simulink model "DSF_A3"  (R2022b)
settings: configuration reference "CommonModelConfiguration" (kept outside this file)
undefined symbols (not defined in the file or in its folder): AccSts1, AdjSpdLimnMsg1, AdjSpdLimnSts2, AdjSpdLimnWarnCoding, AsyLaneChgPsbl1, AsyLaneChgSts2, AsyLaneChgTyp2, AvlStsForAsyLaneChg, AvlStsForLatAutDrv5, AvlStsForLongAutDrv4, AvlStsForSteerSpprt1, Boolean, CarModSts1, CllsnAidPostEve3, CrsCtrlrMsg1, CrsCtrlrSts1, CrvtSpdAdj2, CtryForRoadSgn1, DrvrSpprtFct, E_CommonStatus, E_DSF_Event, E_DSF_Messages, E_DSF_Value, FctSts2, FctStsSpdCtrl, HmiAutnmsSts1, LaneDetnSts1, LCFG_SetSpeedMinKPH, LCFG_SetSpeedMinKPH_A3, LvlWarn1, MplLvlVisWarn1, NoYesCrit1, OffOnNotAvlSrvRqrd, OnOff1, PsdNotPsd, SetSpdSelnForAutDrv1, SpdAdjmtEveForAutDrv, SpdUnit1, SteerIntvSts1, SteerStsForAutDrv3, SteerWarnReqForAutDrv1, SteerWarnSts1, UndrtknPrevnWarnReq, UsgModSts1, VehDetd1, VehSpdIndcdUnit, VisWarnReq1
libraries: simulink x127
(part 2 of 3)

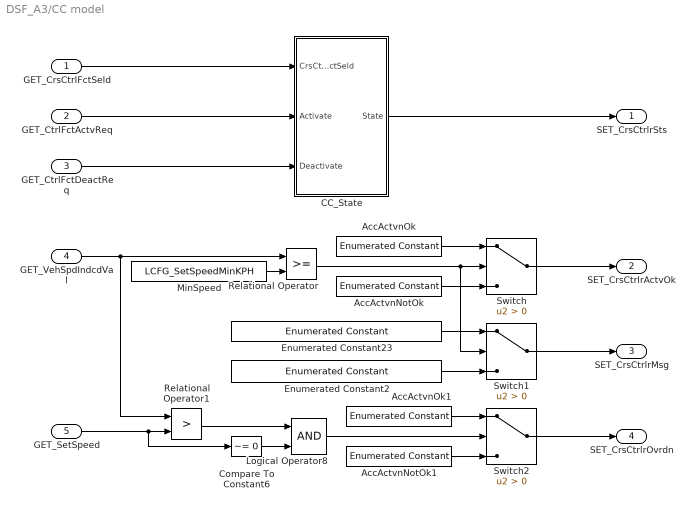
== system DSF_A3/CC model ==
  GET_CrsCtrlFctSeld : Inport
  GET_CtrlFctActvReq : Inport  Port=2
  GET_CtrlFctDeactReq : Inport  Port=3
  GET_VehSpdIndcdVal : Inport  Port=4
  GET_SetSpeed : Inport  Port=5
  AccActvnNotOk : simulink/Sources/Enumerated Constant  OutDataTypeStr=Enum: OnOff1  Value=OnOff1.OnOff1_Off  SampleTime=inf
  AccActvnNotOk1 : simulink/Sources/Enumerated Constant  OutDataTypeStr=Enum: OnOff1  Value=OnOff1.OnOff1_Off  SampleTime=inf
  AccActvnOk : simulink/Sources/Enumerated Constant  OutDataTypeStr=Enum: OnOff1  Value=OnOff1.OnOff1_On  SampleTime=inf
  AccActvnOk1 : simulink/Sources/Enumerated Constant  OutDataTypeStr=Enum: OnOff1  Value=OnOff1.OnOff1_On  SampleTime=inf
  CC_State : Stateflow chart  TreatAsAtomicUnit=on
  Compare To Constant6 : simulink/Logic and Bit Operations/Compare To Constant  relop=~=  const=0  OutDataTypeStr=boolean
  Enumerated Constant2 : simulink/Sources/Enumerated Constant  OutDataTypeStr=Enum: CrsCtrlrMsg1  Value=CrsCtrlrMsg1.CrsCtrlrMsg1_SpdLoLimExcdd  SampleTime=inf
  Enumerated Constant23 : simulink/Sources/Enumerated Constant  OutDataTypeStr=Enum: CrsCtrlrMsg1  Value=CrsCtrlrMsg1.CrsCtrlrMsg1_NoMsg  SampleTime=inf
  Logical Operator8 : Logic  AllPortsSameDT=off  OutDataTypeStr=boolean
  MinSpeed : Constant  Value=LCFG_SetSpeedMinKPH
  Relational Operator : RelationalOperator  OutDataTypeStr=boolean  RndMeth=Simplest  InputSameDT=off
  Relational Operator1 : RelationalOperator  Operator=>  OutDataTypeStr=boolean  RndMeth=Simplest  InputSameDT=off
  Switch : Switch  Criteria=u2 > Threshold  SaturateOnIntegerOverflow=off  InputSameDT=off
  Switch1 : Switch  Criteria=u2 > Threshold  SaturateOnIntegerOverflow=off  InputSameDT=off
  Switch2 : Switch  Criteria=u2 > Threshold  SaturateOnIntegerOverflow=off  InputSameDT=off
  SET_CrsCtrlrSts : Outport
  SET_CrsCtrlrActvOk : Outport  Port=2
  SET_CrsCtrlrMsg : Outport  Port=3
  SET_CrsCtrlrOvrdn : Outport  Port=4
  wires:
  AccActvnOk/1 -> Switch/1
  Relational Operator/1 -> Switch1/2, Switch/2
  MinSpeed/1 -> Relational Operator/2
  GET_VehSpdIndcdVal/1 -> Relational Operator1/1, Relational Operator/1
  Switch/1 -> SET_CrsCtrlrActvOk/1
  AccActvnNotOk/1 -> Switch/3
  Switch1/1 -> SET_CrsCtrlrMsg/1
  Enumerated Constant23/1 -> Switch1/1
  Enumerated Constant2/1 -> Switch1/3
  Switch2/1 -> SET_CrsCtrlrOvrdn/1
  AccActvnOk1/1 -> Switch2/1
  AccActvnNotOk1/1 -> Switch2/3
  Relational Operator1/1 -> Logical Operator8/1
  GET_SetSpeed/1 -> Compare To Constant6/1, Relational Operator1/2
  Logical Operator8/1 -> Switch2/2
  Compare To Constant6/1 -> Logical Operator8/2
  CC_State/1(State) -> SET_CrsCtrlrSts/1
  GET_CrsCtrlFctSeld/1 -> CC_State/1(CrsCtrlFctSeld)
  GET_CtrlFctActvReq/1 -> CC_State/2(Activate)
  GET_CtrlFctDeactReq/1 -> CC_State/3(Deactivate)

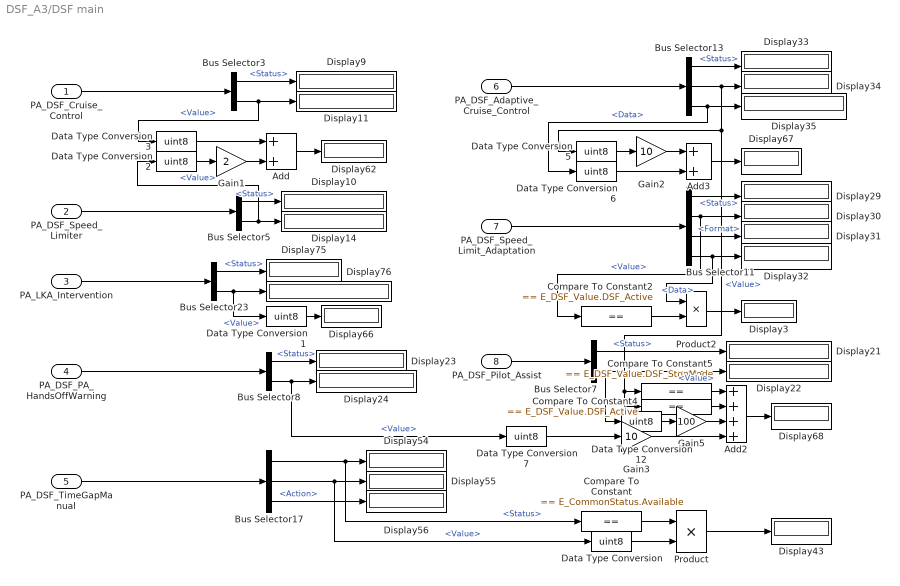
== system DSF_A3/DSF main ==
  PA_DSF_Cruise_Control : Inport
  PA_DSF_Speed_Limiter : Inport  Port=2
  PA_LKA_Intervention : Inport  Port=3
  PA_DSF_PA_HandsOffWarning : Inport  Port=4
  PA_DSF_TimeGapManual : Inport  Port=5
  PA_DSF_Adaptive_Cruise_Control : Inport  Port=6
  PA_DSF_Speed_Limit_Adaptation : Inport  Port=7
  PA_DSF_Pilot_Assist : Inport  Port=8
  Add : Sum
  Add2 : Sum  Inputs=++++
  Add3 : Sum
  Bus Selector11 : BusSelector  OutputSignals=Status,Value,Format,Data
  Bus Selector13 : BusSelector  OutputSignals=Status,Value,Data
  Bus Selector17 : BusSelector  OutputSignals=Status,Value,Action
  Bus Selector{3,5,7..8,23} (5 alike) : BusSelector  OutputSignals=Status,Value
  Compare To Constant : simulink/Logic and Bit Operations/Compare To Constant  relop===  const=E_CommonStatus.Available  OutDataTypeStr=boolean
  Compare To Constant2 : simulink/Logic and Bit Operations/Compare To Constant  relop===  const=E_DSF_Value.DSF_Active  OutDataTypeStr=boolean
  Compare To Constant4 : simulink/Logic and Bit Operations/Compare To Constant  relop===  const=E_DSF_Value.DSF_Active  OutDataTypeStr=boolean
  Compare To Constant5 : simulink/Logic and Bit Operations/Compare To Constant  relop===  const=E_DSF_Value.DSF_StopMode  OutDataTypeStr=boolean
  Data Type Conversion{,1..3,5..7,12} (8 alike) : DataTypeConversion  OutDataTypeStr=uint8  SaturateOnIntegerOverflow=off  RndMeth=Floor
  Display{3,9..11,14,21..24,29..35,43,54..56,62,66..68,75..76} (26 alike) : Display
  Gain1 : Gain  Gain=2
  Gain2 : Gain  Gain=10
  Gain3 : Gain  Gain=10
  Gain5 : Gain  Gain=100
  Product : Product
  Product2 : Product
  wires:
  Add3/1 -> Display67/1
  Bus Selector3/2 -> Data Type Conversion3/1, Display11/1  "<Value>"
  Compare To Constant/1 -> Product/1
  Compare To Constant4/1 -> Add2/2
  Add/1 -> Display62/1
  Product/1 -> Display43/1
  Bus Selector11/3 -> Display31/1  "<Format>"
  Bus Selector11/2 -> Compare To Constant2/1, Display30/1  "<Value>"
  Data Type Conversion12/1 -> Gain5/1
  Gain3/1 -> Add2/4
  Bus Selector17/2 -> Data Type Conversion/1, Display55/1  "<Value>"
  Bus Selector11/4 -> Product2/1, Display32/1  "<Data>"
  Bus Selector7/2 -> Data Type Conversion12/1, Display22/1  "<Value>"
  Data Type Conversion7/1 -> Gain3/1
  Bus Selector23/2 -> Data Type Conversion1/1, Display76/1  "<Value>"
  Bus Selector5/1 -> Display10/1  "<Status>"
  PA_DSF_Cruise_Control/1 -> Bus Selector3/1
  PA_DSF_Speed_Limit_Adaptation/1 -> Bus Selector11/1
  Bus Selector8/2 -> Data Type Conversion7/1, Display24/1  "<Value>"
  Bus Selector13/2 -> Compare To Constant5/1, Compare To Constant4/1, Data Type Conversion5/1, Display34/1  "<Value>"
  Bus Selector13/3 -> Data Type Conversion6/1, Display35/1  "<Data>"
  PA_DSF_Pilot_Assist/1 -> Bus Selector7/1
  Add2/1 -> Display68/1
  Bus Selector5/2 -> Data Type Conversion2/1, Display14/1  "<Value>"
  Bus Selector8/1 -> Display23/1  "<Status>"
  Gain1/1 -> Add/2
  PA_DSF_Adaptive_Cruise_Control/1 -> Bus Selector13/1
  Data Type Conversion1/1 -> Display66/1
  PA_DSF_TimeGapManual/1 -> Bus Selector17/1
  Data Type Conversion3/1 -> Add/1
  Bus Selector7/1 -> Display21/1  "<Status>"
  Bus Selector17/1 -> Compare To Constant/1, Display54/1  "<Status>"
  Bus Selector17/3 -> Display56/1  "<Action>"
  Data Type Conversion5/1 -> Gain2/1
  Bus Selector23/1 -> Display75/1  "<Status>"
  Data Type Conversion6/1 -> Add3/2
  Gain2/1 -> Add3/1
  Product2/1 -> Display3/1
  Compare To Constant2/1 -> Product2/2
  Gain5/1 -> Add2/3
  Compare To Constant5/1 -> Add2/1
  Data Type Conversion2/1 -> Gain1/1
  Bus Selector3/1 -> Display9/1  "<Status>"
  PA_DSF_Speed_Limiter/1 -> Bus Selector5/1
  Bus Selector11/1 -> Display29/1  "<Status>"
  Bus Selector13/1 -> Display33/1  "<Status>"
  Data Type Conversion/1 -> Product/2
  PA_LKA_Intervention/1 -> Bus Selector23/1
  PA_DSF_PA_HandsOffWarning/1 -> Bus Selector8/1

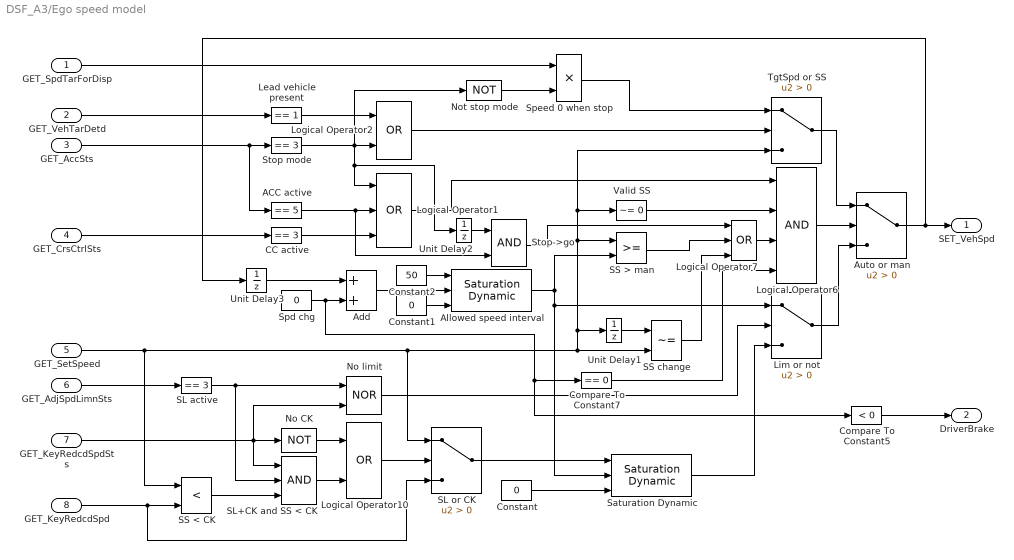
== system DSF_A3/Ego speed model ==
  GET_SpdTarForDisp : Inport
  GET_VehTarDetd : Inport  Port=2
  GET_AccSts : Inport  Port=3
  GET_CrsCtrlSts : Inport  Port=4
  GET_SetSpeed : Inport  Port=5
  GET_AdjSpdLimnSts : Inport  Port=6
  GET_KeyRedcdSpdSts : Inport  Port=7
  GET_KeyRedcdSpd : Inport  Port=8
  ACC active : simulink/Logic and Bit Operations/Compare To Constant  relop===  const=5  OutDataTypeStr=boolean
  Add : Sum
  Allowed speed interval : simulink/Discontinuities/Saturation Dynamic  OutMin=0  OutMax=[]  OutDataTypeStr=Inherit: Same as second input  OutDataType=fixdt(1, 16)  OutScaling=2^-10  DoSatur=off
  Auto or man : Switch  Criteria=u2 > Threshold  SaturateOnIntegerOverflow=off  InputSameDT=off
  CC active : simulink/Logic and Bit Operations/Compare To Constant  relop===  const=3  OutDataTypeStr=boolean
  Compare To Constant5 : simulink/Logic and Bit Operations/Compare To Constant  relop=<  const=0  OutDataTypeStr=boolean
  Compare To Constant7 : simulink/Logic and Bit Operations/Compare To Constant  relop===  const=0  OutDataTypeStr=boolean
  Constant : Constant  Value=0
  Constant1 : Constant  Value=0
  Constant2 : Constant  Value=50
  Lead vehicle present : simulink/Logic and Bit Operations/Compare To Constant  relop===  const=1  OutDataTypeStr=boolean
  Lim or not : Switch  Criteria=u2 > Threshold  SaturateOnIntegerOverflow=off  InputSameDT=off
  Logical Operator1 : Logic  Operator=OR  Inputs=3  AllPortsSameDT=off  OutDataTypeStr=boolean
  Logical Operator10 : Logic  Operator=OR  AllPortsSameDT=off  OutDataTypeStr=boolean
  Logical Operator2 : Logic  Operator=OR  AllPortsSameDT=off  OutDataTypeStr=boolean
  Logical Operator6 : Logic  Inputs=4  AllPortsSameDT=off  OutDataTypeStr=boolean
  Logical Operator7 : Logic  Operator=OR  Inputs=3  AllPortsSameDT=off  OutDataTypeStr=boolean
  No CK : Logic  Operator=NOT  AllPortsSameDT=off  OutDataTypeStr=boolean
  No limit : Logic  Operator=NOR  AllPortsSameDT=off  OutDataTypeStr=boolean
  Not stop mode : Logic  Operator=NOT  AllPortsSameDT=off  OutDataTypeStr=boolean
  SL active : simulink/Logic and Bit Operations/Compare To Constant  relop===  const=3  OutDataTypeStr=boolean
  SL or CK : Switch  Criteria=u2 > Threshold  SaturateOnIntegerOverflow=off  InputSameDT=off
  SL+CK and SS < CK : Logic  Inputs=3  AllPortsSameDT=off  OutDataTypeStr=boolean
  SS < CK : RelationalOperator  Operator=<  OutDataTypeStr=boolean  RndMeth=Simplest  InputSameDT=off
  SS > man : RelationalOperator  OutDataTypeStr=boolean  RndMeth=Simplest  InputSameDT=off
  SS change : RelationalOperator  Operator=~=  OutDataTypeStr=boolean  RndMeth=Simplest  InputSameDT=off
  Saturation Dynamic : simulink/Discontinuities/Saturation Dynamic  OutMin=0  OutMax=[]  OutDataTypeStr=Inherit: Same as second input  OutDataType=fixdt(1, 16)  OutScaling=2^-10  DoSatur=off
  Spd chg : Constant  Value=0  OutDataTypeStr=double
  Speed 0 when stop : Product
  Stop mode : simulink/Logic and Bit Operations/Compare To Constant  relop===  const=3  OutDataTypeStr=boolean
  Stop->go : Logic  AllPortsSameDT=off  OutDataTypeStr=boolean
  TgtSpd or SS : Switch  Criteria=u2 > Threshold  SaturateOnIntegerOverflow=off  InputSameDT=off
  Unit Delay1 : UnitDelay  InitialCondition=100  SampleTime=-1  HasFrameUpgradeWarning=on
  Unit Delay2 : UnitDelay  InitialCondition=1  SampleTime=-1  HasFrameUpgradeWarning=on
  Unit Delay3 : UnitDelay  InitialCondition=50/3.6  SampleTime=-1  HasFrameUpgradeWarning=on
  Valid SS : simulink/Logic and Bit Operations/Compare To Constant  relop=~=  const=0  OutDataTypeStr=boolean
  SET_VehSpd : Outport
  DriverBrake : Outport  Port=2
  wires:
  Logical Operator2/1 -> TgtSpd or SS/2
  ACC active/1 -> Stop->go/2, Logical Operator1/2
  Logical Operator10/1 -> SL or CK/2
  CC active/1 -> Logical Operator1/3
  GET_CrsCtrlSts/1 -> CC active/1
  SL+CK and SS < CK/1 -> Logical Operator10/2
  Lim or not/1 -> Auto or man/3
  GET_SpdTarForDisp/1 -> Speed 0 when stop/1
  Spd chg/1 -> Compare To Constant5/1, Compare To Constant7/1, Add/2
  Logical Operator1/1 -> Logical Operator6/1
  SS > man/1 -> Logical Operator7/2
  Saturation Dynamic/1 -> Lim or not/3
  Constant/1 -> Saturation Dynamic/3
  GET_KeyRedcdSpd/1 -> SL or CK/3, SS < CK/2
  Speed 0 when stop/1 -> TgtSpd or SS/1
  Stop->go/1 -> Logical Operator7/1
  Allowed speed interval/1 -> Lim or not/1, Saturation Dynamic/2, SS > man/2
  GET_VehTarDetd/1 -> Lead vehicle present/1
  Constant1/1 -> Allowed speed interval/3
  Constant2/1 -> Allowed speed interval/1
  SL or CK/1 -> Saturation Dynamic/1
  Not stop mode/1 -> Speed 0 when stop/2
  Auto or man/1 -> SET_VehSpd/1, Unit Delay3/1
  Unit Delay1/1 -> SS change/1
  Stop mode/1 -> Logical Operator1/1, Unit Delay2/1, Logical Operator2/2, Not stop mode/1
  Add/1 -> Allowed speed interval/2
  Lead vehicle present/1 -> Logical Operator2/1
  SL active/1 -> SL+CK and SS < CK/2, No limit/1
  Unit Delay3/1 -> Add/1
  GET_SetSpeed/1 -> SS < CK/1, SL or CK/1, SS change/2, Unit Delay1/1, TgtSpd or SS/3, Valid SS/1, SS > man/1
  Logical Operator6/1 -> Auto or man/2
  Valid SS/1 -> Logical Operator6/2
  TgtSpd or SS/1 -> Auto or man/1
  GET_AccSts/1 -> ACC active/1, Stop mode/1
  No limit/1 -> Lim or not/2
  Unit Delay2/1 -> Stop->go/1
  Compare To Constant5/1 -> DriverBrake/1
  SS < CK/1 -> SL+CK and SS < CK/3
  SS change/1 -> Logical Operator7/3
  Compare To Constant7/1 -> Logical Operator6/4
  Logical Operator7/1 -> Logical Operator6/3
  No CK/1 -> Logical Operator10/1
  GET_KeyRedcdSpdSts/1 -> SL+CK and SS < CK/1, No CK/1, No limit/2
  GET_AdjSpdLimnSts/1 -> SL active/1

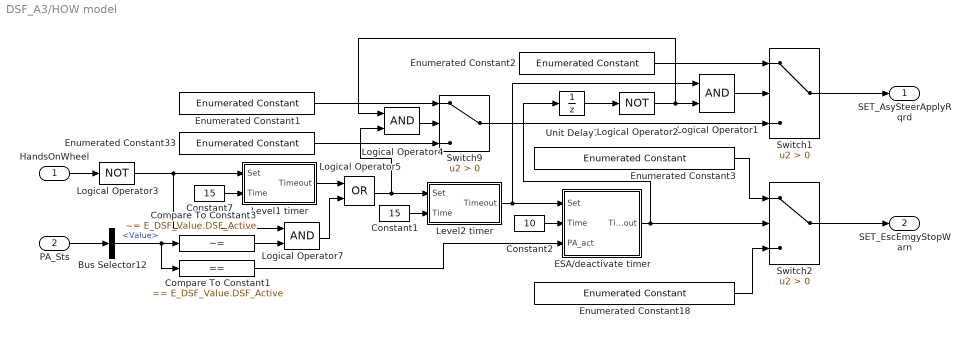
== system DSF_A3/HOW model ==
  HandsOnWheel : Inport
  PA_Sts : Inport  Port=2
  Bus Selector12 : BusSelector  OutputSignals=Value
  Compare To Constant1 : simulink/Logic and Bit Operations/Compare To Constant  relop===  const=E_DSF_Value.DSF_Active  OutDataTypeStr=boolean
  Compare To Constant3 : simulink/Logic and Bit Operations/Compare To Constant  relop=~=  const=E_DSF_Value.DSF_Active  OutDataTypeStr=boolean
  Constant1 : Constant  Value=15
  Constant2 : Constant  Value=10
  Constant7 : Constant  Value=15
  ESA/deactivate timer : Stateflow chart  TreatAsAtomicUnit=on
  Enumerated Constant1 : simulink/Sources/Enumerated Constant  OutDataTypeStr=Enum: LvlWarn1  Value=LvlWarn1.LvlWarn1_Lvl1  SampleTime=inf
  Enumerated Constant18 : simulink/Sources/Enumerated Constant  OutDataTypeStr=Enum: MplLvlVisWarn1  Value=MplLvlVisWarn1.MplLvlVisWarn1_Off  SampleTime=inf
  Enumerated Constant2 : simulink/Sources/Enumerated Constant  OutDataTypeStr=Enum: LvlWarn1  Value=LvlWarn1.LvlWarn1_Lvl2  SampleTime=inf
  Enumerated Constant3 : simulink/Sources/Enumerated Constant  OutDataTypeStr=Enum: MplLvlVisWarn1  Value=MplLvlVisWarn1.MplLvlVisWarn1_WarnLvl1  SampleTime=inf
  Enumerated Constant33 : simulink/Sources/Enumerated Constant  OutDataTypeStr=Enum: LvlWarn1  Value=LvlWarn1.LvlWarn1_NoWarn  SampleTime=inf
  Level1 timer : Stateflow chart  TreatAsAtomicUnit=on
  Level2 timer : Stateflow chart  TreatAsAtomicUnit=on
  Logical Operator1 : Logic  AllPortsSameDT=off  OutDataTypeStr=boolean
  Logical Operator2 : Logic  Operator=NOT  AllPortsSameDT=off  OutDataTypeStr=boolean
  Logical Operator3 : Logic  Operator=NOT  AllPortsSameDT=off  OutDataTypeStr=boolean
  Logical Operator4 : Logic  AllPortsSameDT=off  OutDataTypeStr=boolean
  Logical Operator5 : Logic  Operator=OR  AllPortsSameDT=off  OutDataTypeStr=boolean
  Logical Operator7 : Logic  AllPortsSameDT=off  OutDataTypeStr=boolean
  Switch1 : Switch  Criteria=u2 > Threshold  SaturateOnIntegerOverflow=off  InputSameDT=off
  Switch2 : Switch  Criteria=u2 > Threshold  SaturateOnIntegerOverflow=off  InputSameDT=off
  Switch9 : Switch  Criteria=u2 > Threshold  SaturateOnIntegerOverflow=off  InputSameDT=off
  Unit Delay7 : UnitDelay  InitialCondition=70  SampleTime=-1  HasFrameUpgradeWarning=on
  SET_AsySteerApplyRqrd : Outport
  SET_EscEmgyStopWarn : Outport  Port=2
  wires:
  Constant7/1 -> Level1 timer/2(Time)
  HandsOnWheel/1 -> Logical Operator3/1
  Level1 timer/1(Timeout) -> Logical Operator5/1
  Constant1/1 -> Level2 timer/2(Time)
  Enumerated Constant33/1 -> Switch9/3
  Enumerated Constant1/1 -> Switch9/1
  Switch9/1 -> Switch1/3
  Enumerated Constant2/1 -> Switch1/1
  Switch1/1 -> SET_AsySteerApplyRqrd/1
  Level2 timer/1(Timeout) -> Logical Operator1/1, ESA/deactivate timer/1(Set)
  Constant2/1 -> ESA/deactivate timer/2(Time)
  Enumerated Constant18/1 -> Switch2/3
  Switch2/1 -> SET_EscEmgyStopWarn/1
  Enumerated Constant3/1 -> Switch2/1
  Logical Operator3/1 -> Logical Operator7/1, Level1 timer/1(Set)
  Logical Operator1/1 -> Switch1/2
  Logical Operator2/1 -> Logical Operator4/1, Logical Operator1/2
  Unit Delay7/1 -> Logical Operator2/1
  Logical Operator4/1 -> Switch9/2
  PA_Sts/1 -> Bus Selector12/1
  Bus Selector12/1 -> Compare To Constant1/1, Compare To Constant3/1  "<Value>"
  Compare To Constant3/1 -> Logical Operator7/2
  Logical Operator5/1 -> Logical Operator4/2, Level2 timer/1(Set)
  ESA/deactivate timer/1(Timeout) -> Unit Delay7/1, Switch2/2
  Logical Operator7/1 -> Logical Operator5/2
  Compare To Constant1/1 -> ESA/deactivate timer/3(PA_act)

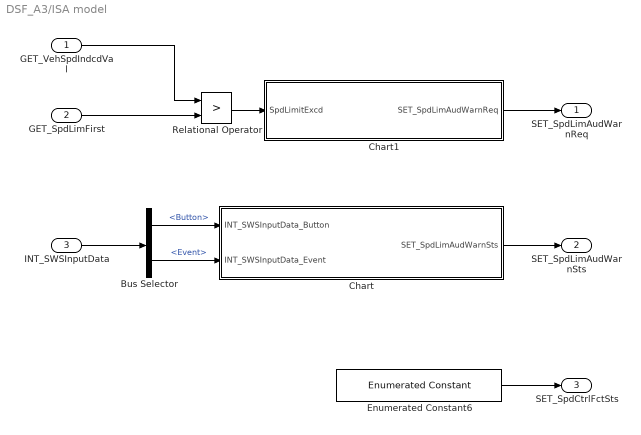
== system DSF_A3/ISA model ==
  GET_VehSpdIndcdVal : Inport
  GET_SpdLimFirst : Inport  Port=2
  INT_SWSInputData : Inport  Port=3
  Bus Selector : BusSelector  OutputSignals=Button,Event
  Chart : Stateflow chart  TreatAsAtomicUnit=on
  Chart1 : Stateflow chart  TreatAsAtomicUnit=on
  Enumerated Constant6 : simulink/Sources/Enumerated Constant  OutDataTypeStr=Enum: FctStsSpdCtrl  Value=FctStsSpdCtrl.FctStsSpdCtrl_Active  SampleTime=inf
  Relational Operator : RelationalOperator  Operator=>  OutDataTypeStr=boolean  RndMeth=Simplest  InputSameDT=off
  SET_SpdLimAudWarnReq : Outport  OutDataTypeStr=Enum: OnOff1
  SET_SpdLimAudWarnSts : Outport  Port=2
  SET_SpdCtrlFctSts : Outport  Port=3
  wires:
  Enumerated Constant6/1 -> SET_SpdCtrlFctSts/1
  INT_SWSInputData/1 -> Bus Selector/1
  Bus Selector/1 -> Chart/1(INT_SWSInputData_Button)  "<Button>"
  Bus Selector/2 -> Chart/2(INT_SWSInputData_Event)  "<Event>"
  Chart/1(SET_SpdLimAudWarnSts) -> SET_SpdLimAudWarnSts/1
  Relational Operator/1 -> Chart1/1(SpdLimitExcd)
  GET_SpdLimFirst/1 -> Relational Operator/2
  Chart1/1(SET_SpdLimAudWarnReq) -> SET_SpdLimAudWarnReq/1
  GET_VehSpdIndcdVal/1 -> Relational Operator/1

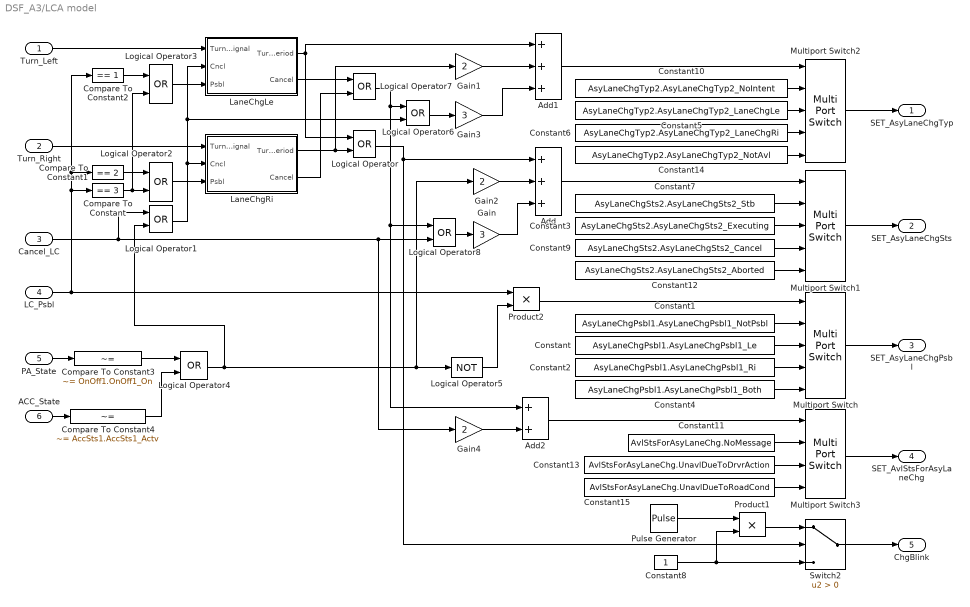
== system DSF_A3/LCA model ==
  Turn_Left : Inport
  Turn_Right : Inport  Port=2
  Cancel_LC : Inport  Port=3
  LC_Psbl : Inport  Port=4
  PA_State : Inport  Port=5
  ACC_State : Inport  Port=6
  Add : Sum  Inputs=+++
  Add1 : Sum  Inputs=+++
  Add2 : Sum
  Compare To Constant : simulink/Logic and Bit Operations/Compare To Constant  relop===  const=3  OutDataTypeStr=boolean
  Compare To Constant1 : simulink/Logic and Bit Operations/Compare To Constant  relop===  const=2  OutDataTypeStr=boolean
  Compare To Constant2 : simulink/Logic and Bit Operations/Compare To Constant  relop===  const=1  OutDataTypeStr=boolean
  Compare To Constant3 : simulink/Logic and Bit Operations/Compare To Constant  relop=~=  const=OnOff1.OnOff1_On  OutDataTypeStr=boolean
  Compare To Constant4 : simulink/Logic and Bit Operations/Compare To Constant  relop=~=  const=AccSts1.AccSts1_Actv  OutDataTypeStr=boolean
  Constant : Constant  Value=AsyLaneChgPsbl1.AsyLaneChgPsbl1_Le
  Constant1 : Constant  Value=AsyLaneChgPsbl1.AsyLaneChgPsbl1_NotPsbl
  Constant10 : Constant  Value=AsyLaneChgTyp2.AsyLaneChgTyp2_NoIntent
  Constant11 : Constant  Value=AvlStsForAsyLaneChg.NoMessage
  Constant12 : Constant  Value=AsyLaneChgSts2.AsyLaneChgSts2_Aborted
  Constant13 : Constant  Value=AvlStsForAsyLaneChg.UnavlDueToDrvrAction
  Constant14 : Constant  Value=AsyLaneChgTyp2.AsyLaneChgTyp2_NotAvl
  Constant15 : Constant  Value=AvlStsForAsyLaneChg.UnavlDueToRoadCond
  Constant2 : Constant  Value=AsyLaneChgPsbl1.AsyLaneChgPsbl1_Ri
  Constant3 : Constant  Value=AsyLaneChgSts2.AsyLaneChgSts2_Executing
  Constant4 : Constant  Value=AsyLaneChgPsbl1.AsyLaneChgPsbl1_Both
  Constant5 : Constant  Value=AsyLaneChgTyp2.AsyLaneChgTyp2_LaneChgLe
  Constant6 : Constant  Value=AsyLaneChgTyp2.AsyLaneChgTyp2_LaneChgRi
  Constant7 : Constant  Value=AsyLaneChgSts2.AsyLaneChgSts2_Stb
  Constant8 : Constant  OutDataTypeStr=uint8
  Constant9 : Constant  Value=AsyLaneChgSts2.AsyLaneChgSts2_Cancel
  Gain : Gain  Gain=3  OutDataTypeStr=uint8
  Gain1 : Gain  Gain=2  OutDataTypeStr=uint8
  Gain2 : Gain  Gain=2  OutDataTypeStr=uint8
  Gain3 : Gain  Gain=3  OutDataTypeStr=uint8
  Gain4 : Gain  Gain=2  OutDataTypeStr=uint8
  LaneChgLe : Stateflow chart  TreatAsAtomicUnit=on
  LaneChgRi : Stateflow chart  TreatAsAtomicUnit=on
  Logical Operator{,1..4,6..8} (8 alike) : Logic  Operator=OR  AllPortsSameDT=off  OutDataTypeStr=boolean
  Logical Operator5 : Logic  Operator=NOT  AllPortsSameDT=off  OutDataTypeStr=boolean
  Multiport Switch : MultiPortSwitch  DataPortOrder=Zero-based contiguous  Inputs=4  DataPortIndices={1,2,3,0}  zeroidx=on  SaturateOnIntegerOverflow=off  InputSameDT=off
  Multiport Switch1 : MultiPortSwitch  DataPortOrder=Zero-based contiguous  Inputs=4  DataPortIndices={1,2,3,0}  DiagnosticForDefault=None  zeroidx=on  SaturateOnIntegerOverflow=off  InputSameDT=off
  Multiport Switch2 : MultiPortSwitch  DataPortOrder=Zero-based contiguous  Inputs=4  DataPortIndices={1,2,3,0}  zeroidx=on  SaturateOnIntegerOverflow=off  InputSameDT=off
  Multiport Switch3 : MultiPortSwitch  DataPortOrder=Zero-based contiguous  DataPortIndices={1,2,3,0}  zeroidx=on  SaturateOnIntegerOverflow=off  InputSameDT=off
  Product1 : Product  OutDataTypeStr=uint8
  Product2 : Product  OutDataTypeStr=uint8
  Pulse Generator : DiscretePulseGenerator  PulseType=Time based  Period=0.5  PulseWidth=50
  Switch2 : Switch  Criteria=u2 > Threshold  SaturateOnIntegerOverflow=off  InputSameDT=off
  SET_AsyLaneChgTyp : Outport
  SET_AsyLaneChgSts : Outport  Port=2
  SET_AsyLaneChgPsbl : Outport  Port=3
  SET_AvlStsForAsyLaneChg : Outport  Port=4
  ChgBlink : Outport  Port=5
  wires:
  Constant/1 -> Multiport Switch/3
  Constant1/1 -> Multiport Switch/2
  Constant2/1 -> Multiport Switch/4
  Constant4/1 -> Multiport Switch/5
  Multiport Switch/1 -> SET_AsyLaneChgPsbl/1
  LC_Psbl/1 -> Product2/1, Compare To Constant2/1, Compare To Constant1/1, Compare To Constant/1
  Multiport Switch1/1 -> SET_AsyLaneChgSts/1
  Constant3/1 -> Multiport Switch1/3
  Constant7/1 -> Multiport Switch1/2
  Logical Operator/1 -> Switch2/2, Add/1
  Turn_Right/1 -> LaneChgRi/1(TurnSignal)
  Turn_Left/1 -> LaneChgLe/1(TurnSignal)
  Constant6/1 -> Multiport Switch2/4
  Constant5/1 -> Multiport Switch2/3
  Product1/1 -> Switch2/1
  Pulse Generator/1 -> Product1/1
  Switch2/1 -> ChgBlink/1
  Constant8/1 -> Product1/2, Switch2/3
  LaneChgLe/1(TurnPeriod) -> Logical Operator/1, Add1/1
  LaneChgRi/1(TurnPeriod) -> Gain1/1, Logical Operator/2
  Constant9/1 -> Multiport Switch1/4
  Cancel_LC/1 -> Gain4/1, Logical Operator8/2, Logical Operator1/1
  Gain/1 -> Add/3
  Multiport Switch2/1 -> SET_AsyLaneChgTyp/1
  Constant10/1 -> Multiport Switch2/2
  Add1/1 -> Multiport Switch2/1
  Gain1/1 -> Add1/2
  Constant11/1 -> Multiport Switch3/2
  Constant12/1 -> Multiport Switch1/5
  Add/1 -> Multiport Switch1/1
  Logical Operator2/1 -> LaneChgRi/3(Psbl)
  Compare To Constant1/1 -> Logical Operator2/1
  Compare To Constant/1 -> Logical Operator3/2, Logical Operator2/2
  Compare To Constant2/1 -> Logical Operator3/1
  Logical Operator3/1 -> LaneChgLe/3(Psbl)
  Constant13/1 -> Multiport Switch3/3
  Multiport Switch3/1 -> SET_AvlStsForAsyLaneChg/1
  Gain2/1 -> Add/2
  Compare To Constant3/1 -> Logical Operator4/1
  ACC_State/1 -> Compare To Constant4/1
  Compare To Constant4/1 -> Logical Operator4/2
  Logical Operator4/1 -> Logical Operator1/2, Logical Operator5/1, Gain2/1
  PA_State/1 -> Compare To Constant3/1
  Logical Operator1/1 -> LaneChgRi/2(Cncl), LaneChgLe/2(Cncl), Logical Operator6/2
  Constant14/1 -> Multiport Switch2/5
  Gain3/1 -> Add1/3
  Product2/1 -> Multiport Switch/1
  Logical Operator5/1 -> Product2/2
  LaneChgLe/2(Cancel) -> Logical Operator7/1
  LaneChgRi/2(Cancel) -> Logical Operator7/2
  Logical Operator6/1 -> Gain3/1
  Logical Operator7/1 -> Add2/1, Logical Operator8/1, Logical Operator6/1
  Logical Operator8/1 -> Gain/1
  Add2/1 -> Multiport Switch3/1
  Gain4/1 -> Add2/2
  Constant15/1 -> Multiport Switch3/4

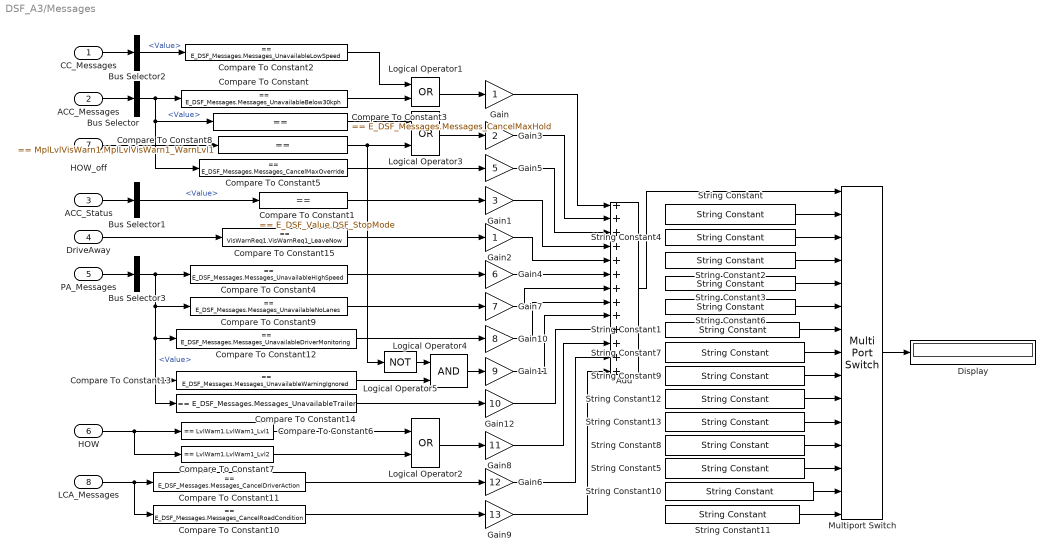
== system DSF_A3/Messages ==
  CC_Messages : Inport
  ACC_Messages : Inport  Port=2
  ACC_Status : Inport  Port=3
  DriveAway : Inport  Port=4
  PA_Messages : Inport  Port=5
  HOW : Inport  Port=6
  HOW_off : Inport  Port=7
  LCA_Messages : Inport  Port=8
  Add : Sum  Inputs=+++++++++++++  InputSameDT=on  OutDataTypeStr=uint8
  Bus Selector{,1..3} (4 alike) : BusSelector  OutputSignals=Value
  Compare To Constant : simulink/Logic and Bit Operations/Compare To Constant  relop===  const=E_DSF_Messages.Messages_UnavailableBelow30kph  OutDataTypeStr=boolean
  Compare To Constant1 : simulink/Logic and Bit Operations/Compare To Constant  relop===  const=E_DSF_Value.DSF_StopMode  OutDataTypeStr=boolean
  Compare To Constant10 : simulink/Logic and Bit Operations/Compare To Constant  relop===  const=E_DSF_Messages.Messages_CancelRoadCondition  OutDataTypeStr=boolean
  Compare To Constant11 : simulink/Logic and Bit Operations/Compare To Constant  relop===  const=E_DSF_Messages.Messages_CancelDriverAction  OutDataTypeStr=boolean
  Compare To Constant12 : simulink/Logic and Bit Operations/Compare To Constant  relop===  const=E_DSF_Messages.Messages_UnavailableDriverMonitoring  OutDataTypeStr=boolean
  Compare To Constant13 : simulink/Logic and Bit Operations/Compare To Constant  relop===  const=E_DSF_Messages.Messages_UnavailableWarningIgnored  OutDataTypeStr=boolean
  Compare To Constant14 : simulink/Logic and Bit Operations/Compare To Constant  relop===  const=E_DSF_Messages.Messages_UnavailableTrailer  OutDataTypeStr=boolean
  Compare To Constant15 : simulink/Logic and Bit Operations/Compare To Constant  relop===  const=VisWarnReq1.VisWarnReq1_LeaveNow  OutDataTypeStr=boolean
  Compare To Constant2 : simulink/Logic and Bit Operations/Compare To Constant  relop===  const=E_DSF_Messages.Messages_UnavailableLowSpeed  OutDataTypeStr=boolean
  Compare To Constant3 : simulink/Logic and Bit Operations/Compare To Constant  relop===  const=E_DSF_Messages.Messages_CancelMaxHold  OutDataTypeStr=boolean
  Compare To Constant4 : simulink/Logic and Bit Operations/Compare To Constant  relop===  const=E_DSF_Messages.Messages_UnavailableHighSpeed  OutDataTypeStr=boolean
  Compare To Constant5 : simulink/Logic and Bit Operations/Compare To Constant  relop===  const=E_DSF_Messages.Messages_CancelMaxOverride  OutDataTypeStr=boolean
  Compare To Constant6 : simulink/Logic and Bit Operations/Compare To Constant  relop===  const=LvlWarn1.LvlWarn1_Lvl1  OutDataTypeStr=boolean
  Compare To Constant7 : simulink/Logic and Bit Operations/Compare To Constant  relop===  const=LvlWarn1.LvlWarn1_Lvl2  OutDataTypeStr=boolean
  Compare To Constant8 : simulink/Logic and Bit Operations/Compare To Constant  relop===  const=MplLvlVisWarn1.MplLvlVisWarn1_WarnLvl1  OutDataTypeStr=boolean
  Compare To Constant9 : simulink/Logic and Bit Operations/Compare To Constant  relop===  const=E_DSF_Messages.Messages_UnavailableNoLanes  OutDataTypeStr=boolean
  Display : Display
  Gain : Gain  OutDataTypeStr=uint8
  Gain1 : Gain  Gain=3  OutDataTypeStr=uint8
  Gain10 : Gain  Gain=8  OutDataTypeStr=uint8
  Gain11 : Gain  Gain=9  OutDataTypeStr=uint8
  Gain12 : Gain  Gain=10  OutDataTypeStr=uint8
  Gain2 : Gain  OutDataTypeStr=uint8
  Gain3 : Gain  Gain=2  OutDataTypeStr=uint8
  Gain4 : Gain  Gain=6  OutDataTypeStr=uint8
  Gain5 : Gain  Gain=5  OutDataTypeStr=uint8
  Gain6 : Gain  Gain=12  OutDataTypeStr=uint8
  Gain7 : Gain  Gain=7  OutDataTypeStr=uint8
  Gain8 : Gain  Gain=11  OutDataTypeStr=uint8
  Gain9 : Gain  Gain=13  OutDataTypeStr=uint8
  Logical Operator1 : Logic  Operator=OR  AllPortsSameDT=off  OutDataTypeStr=boolean
  Logical Operator2 : Logic  Operator=OR  AllPortsSameDT=off  OutDataTypeStr=boolean
  Logical Operator3 : Logic  Operator=OR  AllPortsSameDT=off  OutDataTypeStr=boolean
  Logical Operator4 : Logic  AllPortsSameDT=off  OutDataTypeStr=boolean
  Logical Operator5 : Logic  Operator=NOT  AllPortsSameDT=off  OutDataTypeStr=boolean
  Multiport Switch : MultiPortSwitch  DataPortOrder=Specify indices  Inputs=4  DataPortIndices={1,2,3,4,5,6,7,8,9,10,11,12,13,14}  DiagnosticForDefault=None  OutDataTypeStr=string  SaturateOnIntegerOverflow=off
  String Constant : StringConstant  String="\"Unavailable speed too low\""
  String Constant1 : StringConstant  String="\"Unavailable speed too high\""
  String Constant10 : StringConstant  String="\"Lane change cancel road cond\""
  String Constant11 : StringConstant  String="\"\""
  String Constant12 : StringConstant  String="\"Warning ignored\""
  String Constant13 : StringConstant  String="\"Trailer connected\""
  String Constant2 : StringConstant  String="\"Press resume to drive!\""
  String Constant3 : StringConstant  String="\"Ready to drive?\""
  String Constant4 : StringConstant  String="\"Deactivated\""
  String Constant5 : StringConstant  String="\"Lane change cancel by driver\""
  String Constant6 : StringConstant  String="\"Too long manual drive\""
  String Constant7 : StringConstant  String="\"Unavailable no lanes detected\""
  String Constant8 : StringConstant  String="\"Keep hands on steering wheel\""
  String Constant9 : StringConstant  String="\"No driver monitoring\""
  wires:
  ACC_Messages/1 -> Bus Selector/1
  Bus Selector/1 -> Compare To Constant/1, Compare To Constant5/1, Compare To Constant3/1  "<Value>"
  Compare To Constant/1 -> Logical Operator1/2
  String Constant/1 -> Multiport Switch/2
  String Constant1/1 -> Multiport Switch/7
  Multiport Switch/1 -> Display/1
  ACC_Status/1 -> Bus Selector1/1
  Bus Selector1/1 -> Compare To Constant1/1  "<Value>"
  String Constant2/1 -> Multiport Switch/4
  String Constant3/1 -> Multiport Switch/5
  Gain/1 -> Add/1
  Compare To Constant1/1 -> Gain1/1
  Compare To Constant15/1 -> Gain2/1
  Gain1/1 -> Add/4
  Gain2/1 -> Add/5
  Add/1 -> Multiport Switch/1
  DriveAway/1 -> Compare To Constant15/1
  CC_Messages/1 -> Bus Selector2/1
  Bus Selector2/1 -> Compare To Constant2/1  "<Value>"
  Logical Operator1/1 -> Gain/1
  Compare To Constant2/1 -> Logical Operator1/1
  Compare To Constant3/1 -> Logical Operator3/1
  Gain3/1 -> Add/2
  String Constant4/1 -> Multiport Switch/3
  Gain4/1 -> Add/6
  PA_Messages/1 -> Bus Selector3/1
  Compare To Constant4/1 -> Gain4/1
  Compare To Constant5/1 -> Gain5/1
  Gain5/1 -> Add/3
  String Constant6/1 -> Multiport Switch/6
  Compare To Constant6/1 -> Logical Operator2/1
  Compare To Constant7/1 -> Logical Operator2/2
  Logical Operator2/1 -> Gain8/1
  Gain6/1 -> Add/12
  String Constant7/1 -> Multiport Switch/8
  HOW/1 -> Compare To Constant7/1, Compare To Constant6/1
  HOW_off/1 -> Compare To Constant8/1
  Logical Operator3/1 -> Gain3/1
  Compare To Constant8/1 -> Logical Operator5/1, Logical Operator3/2
  Bus Selector3/1 -> Compare To Constant4/1, Compare To Constant9/1, Compare To Constant14/1, Compare To Constant13/1, Compare To Constant12/1  "<Value>"
  Compare To Constant9/1 -> Gain7/1
  Gain7/1 -> Add/7
  Gain8/1 -> Add/11
  LCA_Messages/1 -> Compare To Constant10/1, Compare To Constant11/1
  Compare To Constant11/1 -> Gain6/1
  Compare To Constant10/1 -> Gain9/1
  Gain9/1 -> Add/13
  String Constant11/1 -> Multiport Switch/15
  Gain10/1 -> Add/8
  Compare To Constant12/1 -> Gain10/1
  String Constant10/1 -> Multiport Switch/14
  String Constant8/1 -> Multiport Switch/12
  String Constant5/1 -> Multiport Switch/13
  String Constant9/1 -> Multiport Switch/9
  Compare To Constant13/1 -> Logical Operator4/2
  Gain11/1 -> Add/9
  String Constant12/1 -> Multiport Switch/10
  Logical Operator4/1 -> Gain11/1
  Logical Operator5/1 -> Logical Operator4/1
  Compare To Constant14/1 -> Gain12/1
  Gain12/1 -> Add/10
  String Constant13/1 -> Multiport Switch/11

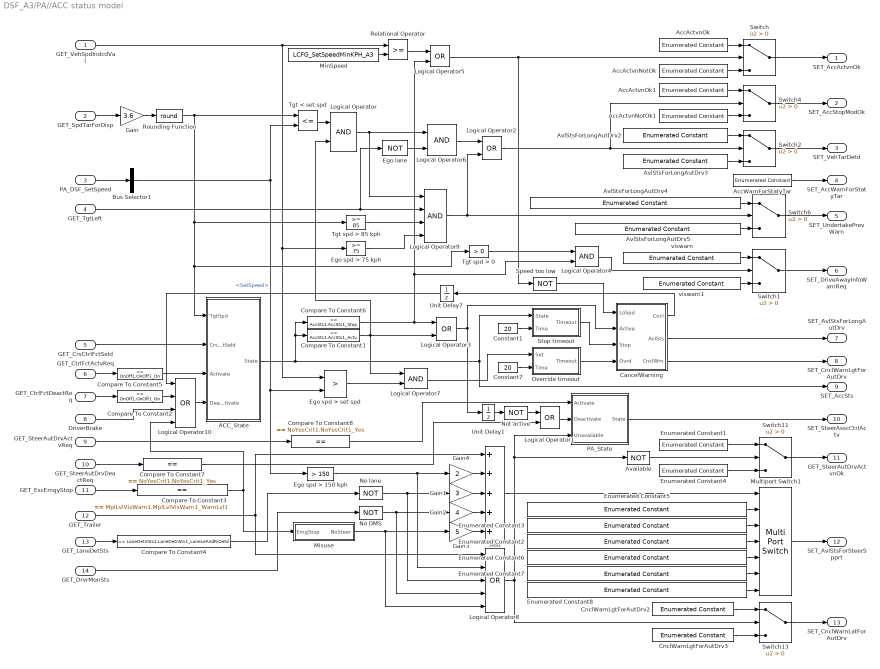
== system DSF_A3/PA//ACC status model ==
  GET_VehSpdIndcdVal : Inport
  GET_SpdTarForDisp : Inport  Port=2
  PA_DSF_SetSpeed : Inport  Port=3
  GET_TgtLeft : Inport  Port=4
  GET_CrsCtrlFctSeld : Inport  Port=5
  GET_CtrlFctActvReq : Inport  Port=6
  GET_CtrlFctDeactReq : Inport  Port=7
  DriverBrake : Inport  Port=8
  GET_SteerAutDrvActvReq : Inport  Port=9
  GET_SteerAutDrvDeactReq : Inport  Port=10
  GET_EscEmgyStop : Inport  Port=11
  GET_Trailer : Inport  Port=12
  GET_LaneDetSts : Inport  Port=13
  GET_DrvrMonSts : Inport  Port=14
  ACC_State : Stateflow chart  TreatAsAtomicUnit=on
  AccActvnNotOk : simulink/Sources/Enumerated Constant  OutDataTypeStr=Enum: OnOff1  Value=OnOff1.OnOff1_Off  SampleTime=inf
  AccActvnNotOk1 : simulink/Sources/Enumerated Constant  OutDataTypeStr=Enum: OnOff1  Value=OnOff1.OnOff1_Off  SampleTime=inf
  AccActvnOk : simulink/Sources/Enumerated Constant  OutDataTypeStr=Enum: OnOff1  Value=OnOff1.OnOff1_On  SampleTime=inf
  AccActvnOk1 : simulink/Sources/Enumerated Constant  OutDataTypeStr=Enum: OnOff1  Value=OnOff1.OnOff1_On  SampleTime=inf
  AccWarnForStatyTar : simulink/Sources/Enumerated Constant  OutDataTypeStr=Enum: OnOff1  Value=OnOff1.OnOff1_Off  SampleTime=inf
  Add : Sum  Inputs=+++++
  Available : Logic  Operator=NOT  AllPortsSameDT=off  OutDataTypeStr=boolean
  AvlStsForLongAutDrv2 : simulink/Sources/Enumerated Constant  OutDataTypeStr=Enum: VehDetd1  Value=VehDetd1.VehDetd1_VehDetdSng  SampleTime=inf
  AvlStsForLongAutDrv3 : simulink/Sources/Enumerated Constant  OutDataTypeStr=Enum: VehDetd1  Value=VehDetd1.VehDetd1_NoVehDetd  SampleTime=inf
  AvlStsForLongAutDrv4 : simulink/Sources/Enumerated Constant  OutDataTypeStr=Enum: UndrtknPrevnWarnReq  Value=UndrtknPrevnWarnReq.UndrtknPrevnWarnReq_WarnForUndrtknPrevnLe  SampleTime=inf
  AvlStsForLongAutDrv5 : simulink/Sources/Enumerated Constant  OutDataTypeStr=Enum: UndrtknPrevnWarnReq  Value=UndrtknPrevnWarnReq.UndrtknPrevnWarnReq_NoWarn  SampleTime=inf
  Bus Selector1 : BusSelector  OutputSignals=SetSpeed
  CancelWarning : Subsystem
  CnclWarnLgtForAutDrv2 : simulink/Sources/Enumerated Constant  OutDataTypeStr=Enum: NoYesCrit1  Value=NoYesCrit1.NoYesCrit1_Yes  SampleTime=inf
  CnclWarnLgtForAutDrv3 : simulink/Sources/Enumerated Constant  OutDataTypeStr=Enum: NoYesCrit1  Value=NoYesCrit1.NoYesCrit1_No  SampleTime=inf
  Compare To Constant1 : simulink/Logic and Bit Operations/Compare To Constant  relop===  const=AccSts1.AccSts1_Actv  OutDataTypeStr=boolean
  Compare To Constant2 : simulink/Logic and Bit Operations/Compare To Constant  relop===  const=OnOff1.OnOff1_On  OutDataTypeStr=boolean
  Compare To Constant3 : simulink/Logic and Bit Operations/Compare To Constant  relop===  const=MplLvlVisWarn1.MplLvlVisWarn1_WarnLvl1  OutDataTypeStr=boolean
  Compare To Constant4 : simulink/Logic and Bit Operations/Compare To Constant  relop===  const=LaneDetnSts1.LaneDetnSts1_LaneLeAndRiDetd  OutDataTypeStr=boolean
  Compare To Constant5 : simulink/Logic and Bit Operations/Compare To Constant  relop===  const=OnOff1.OnOff1_On  OutDataTypeStr=boolean
  Compare To Constant6 : simulink/Logic and Bit Operations/Compare To Constant  relop===  const=AccSts1.AccSts1_Stop  OutDataTypeStr=boolean
  Compare To Constant7 : simulink/Logic and Bit Operations/Compare To Constant  relop===  const=NoYesCrit1.NoYesCrit1_Yes  OutDataTypeStr=boolean
  Compare To Constant8 : simulink/Logic and Bit Operations/Compare To Constant  relop===  const=NoYesCrit1.NoYesCrit1_Yes  OutDataTypeStr=boolean
  Constant1 : Constant  Value=20
  Constant7 : Constant  Value=20
  Ego lane : Logic  Operator=NOT  AllPortsSameDT=off  OutDataTypeStr=boolean
  Ego spd > 150 kph : simulink/Logic and Bit Operations/Compare To Constant  relop=>  const=150  OutDataTypeStr=boolean
  Ego spd > 75 kph : simulink/Logic and Bit Operations/Compare To Constant  relop=>=  const=75  OutDataTypeStr=boolean
  Ego spd > set spd : RelationalOperator  Operator=>  OutDataTypeStr=boolean  RndMeth=Simplest  InputSameDT=off
  Enumerated Constant1 : simulink/Sources/Enumerated Constant  OutDataTypeStr=Enum: OnOff1  Value=OnOff1.OnOff1_On  SampleTime=inf
  Enumerated Constant2 : simulink/Sources/Enumerated Constant  OutDataTypeStr=Enum: AvlStsForSteerSpprt1  Value=AvlStsForSteerSpprt1.AvlStsForSteerSpprt_SteerUnavlSpdTooHigh  SampleTime=inf
  Enumerated Constant3 : simulink/Sources/Enumerated Constant  OutDataTypeStr=Enum: AvlStsForSteerSpprt1  Value=AvlStsForSteerSpprt1.AvlStsForSteerSpprt_SteerUnavlTrailerAttached  SampleTime=inf
  Enumerated Constant4 : simulink/Sources/Enumerated Constant  OutDataTypeStr=Enum: OnOff1  Value=OnOff1.OnOff1_Off  SampleTime=inf
  Enumerated Constant5 : simulink/Sources/Enumerated Constant  OutDataTypeStr=Enum: AvlStsForSteerSpprt1  Value=AvlStsForSteerSpprt1.AvlStsForSteerSpprt_NoMsg  SampleTime=inf
  Enumerated Constant6 : simulink/Sources/Enumerated Constant  OutDataTypeStr=Enum: AvlStsForSteerSpprt1  Value=AvlStsForSteerSpprt1.AvlStsForSteerSpprt_SteerUnavlRoadEstNotPsbl  SampleTime=inf
  Enumerated Constant7 : simulink/Sources/Enumerated Constant  OutDataTypeStr=Enum: AvlStsForSteerSpprt1  Value=AvlStsForSteerSpprt1.AvlStsForSteerSpprt_SteerUnavlDriverMontrUnavail  SampleTime=inf
  Enumerated Constant8 : simulink/Sources/Enumerated Constant  OutDataTypeStr=Enum: AvlStsForSteerSpprt1  Value=AvlStsForSteerSpprt1.AvlStsForSteerSpprt_SteerUnavlRestOfDrive  SampleTime=inf
  Gain : Gain  Gain=3.6  OutDataTypeStr=double
  Gain1 : Gain  Gain=3  OutDataTypeStr=double
  Gain2 : Gain  Gain=4  OutDataTypeStr=double
  Gain3 : Gain  Gain=5  OutDataTypeStr=double
  Gain4 : Gain  Gain=2  OutDataTypeStr=double
  Logical Operator{,4,6..7} (4 alike) : Logic  AllPortsSameDT=off  OutDataTypeStr=boolean
  Logical Operator{1..3,5} (4 alike) : Logic  Operator=OR  AllPortsSameDT=off  OutDataTypeStr=boolean
  Logical Operator10 : Logic  Operator=OR  Inputs=4  AllPortsSameDT=off  OutDataTypeStr=boolean
  Logical Operator8 : Logic  Operator=OR  Inputs=5  AllPortsSameDT=off  OutDataTypeStr=boolean
  Logical Operator9 : Logic  Inputs=4  AllPortsSameDT=off  OutDataTypeStr=boolean
  MinSpeed : Constant  Value=LCFG_SetSpeedMinKPH_A3
  Misuse : Stateflow chart  TreatAsAtomicUnit=on
  Multiport Switch1 : MultiPortSwitch  DataPortOrder=Zero-based contiguous  Inputs=6  DiagnosticForDefault=None  zeroidx=on  SaturateOnIntegerOverflow=off  InputSameDT=off
  No DMS : Logic  Operator=NOT  AllPortsSameDT=off  OutDataTypeStr=boolean
  No lane : Logic  Operator=NOT  AllPortsSameDT=off  OutDataTypeStr=boolean
  Not active : Logic  Operator=NOT  AllPortsSameDT=off  OutDataTypeStr=boolean
  Override timeout : Stateflow chart  TreatAsAtomicUnit=on
  PA_State : Stateflow chart  TreatAsAtomicUnit=on
  Relational Operator : RelationalOperator  OutDataTypeStr=boolean  RndMeth=Simplest  InputSameDT=off
  Rounding Function : Rounding  Operator=round
  Speed too low : Logic  Operator=NOT  AllPortsSameDT=off  OutDataTypeStr=boolean
  Stop timeout : Stateflow chart  TreatAsAtomicUnit=on
  Switch{,1..2,4,6,11,13} (7 alike) : Switch  Criteria=u2 > Threshold  SaturateOnIntegerOverflow=off  InputSameDT=off
  Tgt < set spd : RelationalOperator  Operator=<=  OutDataTypeStr=boolean  RndMeth=Simplest  InputSameDT=off
  Tgt spd > 0 : simulink/Logic and Bit Operations/Compare To Constant  relop=>  const=0  OutDataTypeStr=boolean
  Tgt spd > 85 kph : simulink/Logic and Bit Operations/Compare To Constant  relop=>=  const=85  OutDataTypeStr=boolean
  Unit Delay1 : UnitDelay  SampleTime=-1  HasFrameUpgradeWarning=on
  Unit Delay7 : UnitDelay  SampleTime=-1  HasFrameUpgradeWarning=on
  viswarn : simulink/Sources/Enumerated Constant  OutDataTypeStr=Enum: VisWarnReq1  Value=VisWarnReq1.VisWarnReq1_LeaveNow  SampleTime=inf
  viswarn1 : simulink/Sources/Enumerated Constant  OutDataTypeStr=Enum: VisWarnReq1  Value=VisWarnReq1.VisWarnReq1_Off  SampleTime=inf
  SET_AccActvnOk : Outport
  SET_AccStopModOk : Outport  Port=2
  SET_VehTarDetd : Outport  Port=3
  SET_AccWarnForStatyTar : Outport  Port=4
  SET_UndertakePrevWarn : Outport  Port=5
  SET_DriveAwayInfoWarnReq : Outport  Port=6
  SET_AvlStsForLongAutDrv : Outport  Port=7
  SET_CnclWarnLgtForAutDrv : Outport  Port=8
  SET_AccSts : Outport  Port=9
  SET_SteerAsscCtrlActv : Outport  Port=10
  GET_SteerAutDrvActvnOk : Outport  Port=11
  SET_AvlStsForSteerSpprt : Outport  Port=12
  SET_CnclWarnLatForAutDrv : Outport  Port=13
  wires:
  Switch/1 -> SET_AccActvnOk/1
  AccActvnOk/1 -> Switch/1
  AccActvnNotOk/1 -> Switch/3
  MinSpeed/1 -> Relational Operator/2
  Tgt < set spd/1 -> Logical Operator/1
  Switch2/1 -> SET_VehTarDetd/1
  AvlStsForLongAutDrv2/1 -> Switch2/1
  AvlStsForLongAutDrv3/1 -> Switch2/3
  Compare To Constant1/1 -> Logical Operator/2, Logical Operator7/1, Logical Operator3/2
  GET_SpdTarForDisp/1 -> Gain/1
  Gain/1 -> Rounding Function/1
  AccActvnNotOk1/1 -> Switch4/3
  AccActvnOk1/1 -> Switch4/1
  Switch4/1 -> SET_AccStopModOk/1
  Logical Operator/1 -> Logical Operator9/1, Logical Operator6/1
  Logical Operator2/1 -> Switch4/2, Switch2/2
  Relational Operator/1 -> Logical Operator5/1
  Logical Operator5/1 -> Switch/2, Speed too low/1
  Compare To Constant6/1 -> Logical Operator4/2, Logical Operator5/2, Logical Operator3/1
  AccWarnForStatyTar/1 -> SET_AccWarnForStatyTar/1
  PA_DSF_SetSpeed/1 -> Bus Selector1/1
  Bus Selector1/1 -> Tgt < set spd/2, Ego spd > 150 kph/1, Ego spd > set spd/2  "<SetSpeed>"
  Rounding Function/1 -> Tgt spd > 0/1, ACC_State/1(TgtSpd), Tgt spd > 85 kph/1, Tgt < set spd/1
  Switch6/1 -> SET_UndertakePrevWarn/1
  AvlStsForLongAutDrv5/1 -> Switch6/3
  AvlStsForLongAutDrv4/1 -> Switch6/1
  GET_TgtLeft/1 -> Logical Operator9/2, Ego lane/1
  Logical Operator9/1 -> Switch6/2, Logical Operator2/2
  Override timeout/1(Timeout) -> CancelWarning/4(Ovrd)
  Constant7/1 -> Override timeout/2(Time)
  Ego spd > set spd/1 -> Logical Operator7/2
  Logical Operator7/1 -> Override timeout/1(Set)
  Stop timeout/1(Timeout) -> CancelWarning/3(Stop)
  GET_VehSpdIndcdVal/1 -> Relational Operator/1, Ego spd > set spd/1, Ego spd > 75 kph/1
  Tgt spd > 85 kph/1 -> Logical Operator9/3
  Ego spd > 75 kph/1 -> Logical Operator9/4
  Logical Operator6/1 -> Logical Operator2/1
  Ego lane/1 -> Logical Operator6/2
  Switch11/1 -> GET_SteerAutDrvActvnOk/1
  DriverBrake/1 -> Logical Operator10/3
  Available/1 -> Switch11/2
  GET_LaneDetSts/1 -> Compare To Constant4/1
  Multiport Switch1/1 -> SET_AvlStsForSteerSpprt/1
  Enumerated Constant2/1 -> Multiport Switch1/4
  Enumerated Constant3/1 -> Multiport Switch1/3
  Enumerated Constant5/1 -> Multiport Switch1/2
  Add/1 -> Multiport Switch1/1
  Gain1/1 -> Add/3
  Compare To Constant4/1 -> No lane/1
  Ego spd > 150 kph/1 -> Logical Operator8/2, Gain4/1
  No lane/1 -> Logical Operator8/3, Gain1/1
  Switch13/1 -> SET_CnclWarnLatForAutDrv/1
  CnclWarnLgtForAutDrv3/1 -> Switch13/3
  CnclWarnLgtForAutDrv2/1 -> Switch13/1
  Logical Operator10/1 -> ACC_State/4(Deactivate)
  GET_CtrlFctDeactReq/1 -> Compare To Constant2/1
  GET_CtrlFctActvReq/1 -> Compare To Constant5/1
  GET_CrsCtrlFctSeld/1 -> ACC_State/2(CrsCtrlFctSeld)
  Unit Delay7/1 -> Logical Operator10/1
  GET_EscEmgyStop/1 -> Compare To Constant3/1
  Compare To Constant2/1 -> Logical Operator10/2
  Compare To Constant5/1 -> ACC_State/3(Activate)
  ACC_State/1(State) -> SET_AccSts/1, Stop timeout/1(State), Compare To Constant6/1, Compare To Constant1/1
  Compare To Constant3/1 -> Misuse/1(EmgStop), Logical Operator10/4
  Enumerated Constant4/1 -> Switch11/3
  Enumerated Constant1/1 -> Switch11/1
  PA_State/1(State) -> SET_SteerAsscCtrlActv/1
  Unit Delay1/1 -> Not active/1
  Enumerated Constant6/1 -> Multiport Switch1/5
  GET_DrvrMonSts/1 -> No DMS/1
  Gain2/1 -> Add/4
  No DMS/1 -> Logical Operator8/4, Gain2/1
  Misuse/1(NoSteer) -> Logical Operator8/5, Gain3/1
  Gain3/1 -> Add/5
  Enumerated Constant7/1 -> Multiport Switch1/6
  GET_Trailer/1 -> Logical Operator8/1, Add/1
  Gain4/1 -> Add/2
  Logical Operator8/1 -> Switch13/2, PA_State/3(Unavailable), Available/1
  Enumerated Constant8/1 -> Multiport Switch1/7
  CancelWarning/1(Cncl) -> Unit Delay7/1
  CancelWarning/3(CnclWrn) -> SET_CnclWarnLgtForAutDrv/1
  CancelWarning/2(AvlSts) -> SET_AvlStsForLongAutDrv/1
  Logical Operator3/1 -> Unit Delay1/1, CancelWarning/2(Active)
  Speed too low/1 -> CancelWarning/1(LoSpd)
  Constant1/1 -> Stop timeout/2(Time)
  Switch1/1 -> SET_DriveAwayInfoWarnReq/1
  viswarn/1 -> Switch1/1
  viswarn1/1 -> Switch1/3
  Logical Operator4/1 -> Switch1/2
  Tgt spd > 0/1 -> Logical Operator4/1
  Logical Operator1/1 -> PA_State/2(Deactivate)
  Not active/1 -> Logical Operator1/1
  GET_SteerAutDrvActvReq/1 -> Compare To Constant8/1
  GET_SteerAutDrvDeactReq/1 -> Compare To Constant7/1
  Compare To Constant7/1 -> Logical Operator1/2
  Compare To Constant8/1 -> PA_State/1(Activate)

== system DSF_A3/SL model ==
  GET_DrvrCrsCtrlFctSeld : Inport
  GET_DrvrCrsCtrlFctActvReq : Inport  Port=2
  GET_DrvrCrsCtrlFctDeactvnReq : Inport  Port=3
  GET_CrsCtrlOvrdn : Inport  Port=4
  SL_State : Stateflow chart  TreatAsAtomicUnit=on
  SET_AdjSpdLimnSts : Outport
  wires:
  GET_DrvrCrsCtrlFctSeld/1 -> SL_State/1(CrsCtrlFctSeld)
  SL_State/1(State) -> SET_AdjSpdLimnSts/1
  GET_DrvrCrsCtrlFctDeactvnReq/1 -> SL_State/3(Deactivate)
  GET_DrvrCrsCtrlFctActvReq/1 -> SL_State/2(Activate)
  GET_CrsCtrlOvrdn/1 -> SL_State/4(CrsCtrlOvrdn)

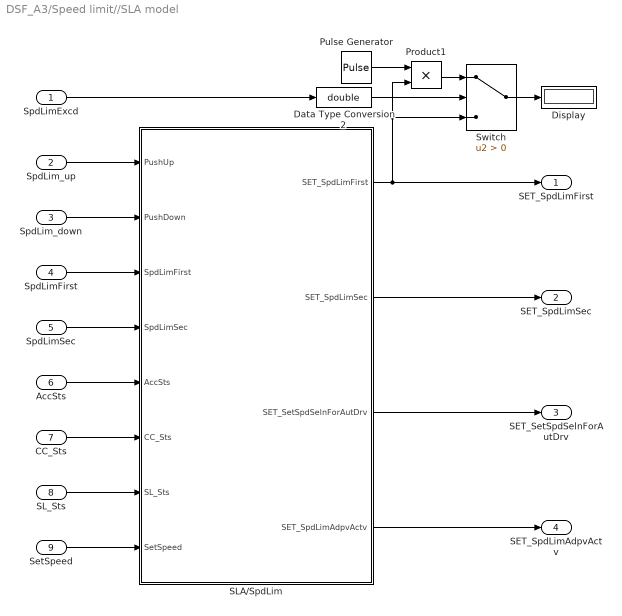
== system DSF_A3/Speed limit//SLA model ==
  SpdLimExcd : Inport
  SpdLim_up : Inport  Port=2
  SpdLim_down : Inport  Port=3
  SpdLimFirst : Inport  Port=4
  SpdLimSec : Inport  Port=5
  AccSts : Inport  Port=6
  CC_Sts : Inport  Port=7
  SL_Sts : Inport  Port=8
  SetSpeed : Inport  Port=9
  Data Type Conversion2 : DataTypeConversion  OutDataTypeStr=double  SaturateOnIntegerOverflow=off  RndMeth=Floor
  Display : Display
  Product1 : Product
  Pulse Generator : DiscretePulseGenerator  PulseType=Time based  Period=0.5  PulseWidth=50
  SLA/SpdLim : Stateflow chart  TreatAsAtomicUnit=on
      settings: PortSchema="{\"entries\":[{\"content\":{\"sides\":[{\"content\":{\"connectorIds\":[\"In1\",\"In2\",\"In3\",\"In4\",\"In5\",\"In6\",\"In7\",\"In8\"]},\"type\":\"ConnectorPlacement.EquallySpacedRectSide\",\"uuid\":\"50a9cfe1-14d0-4131-bd43-42b01cfb3bc1\"},{\"content\":{\"connectorIds\":[\"Out2\",\"Out1\",\"Out3\",\"Out4\"],\"side\":\"RIGHT\"},\"type\":\"ConnectorPlacement.EquallySpacedRectSide\",\"uuid\":\"e893b316-2b3e-4fbb-8898-380048607deb\"},{\"content\":{\"connectorIds\":[],\"side\":\"TOP\"},\"type\":\"ConnectorPlacement.EquallySpacedRectSide\",\"uuid\":\"15802024-6082-4699-9c20-01ccd97957b8\"}]},\"type\":\"ConnectorPlacement.EquallySpacedConnector\",\"uuid\":\"0bbff380-7a2f-4c63-8641-ffef81eb902e\"}],\"packageUris\":[\"http://schema.mathworks.com/mf0/Connector/R2020b\"],\"version\":\"1.0\"}"
  Switch : Switch  Criteria=u2 > Threshold  SaturateOnIntegerOverflow=off  InputSameDT=off
  SET_SpdLimFirst : Outport
  SET_SpdLimSec : Outport  Port=2
  SET_SetSpdSelnForAutDrv : Outport  Port=3
  SET_SpdLimAdpvActv : Outport  Port=4
  wires:
  Data Type Conversion2/1 -> Switch/2
  Pulse Generator/1 -> Product1/1
  SpdLimExcd/1 -> Data Type Conversion2/1
  Switch/1 -> Display/1
  Product1/1 -> Switch/1
  SLA/SpdLim/2(SET_SpdLimFirst) -> SET_SpdLimFirst/1, Product1/2, Switch/3
  SLA/SpdLim/1(SET_SpdLimSec) -> SET_SpdLimSec/1
  SpdLim_down/1 -> SLA/SpdLim/2(PushDown)
  SpdLim_up/1 -> SLA/SpdLim/1(PushUp)
  SpdLimFirst/1 -> SLA/SpdLim/3(SpdLimFirst)
  SpdLimSec/1 -> SLA/SpdLim/4(SpdLimSec)
  SLA/SpdLim/3(SET_SetSpdSelnForAutDrv) -> SET_SetSpdSelnForAutDrv/1
  SLA/SpdLim/4(SET_SpdLimAdpvActv) -> SET_SpdLimAdpvActv/1
  AccSts/1 -> SLA/SpdLim/5(AccSts)
  SetSpeed/1 -> SLA/SpdLim/8(SetSpeed)
  CC_Sts/1 -> SLA/SpdLim/6(CC_Sts)
  SL_Sts/1 -> SLA/SpdLim/7(SL_Sts)

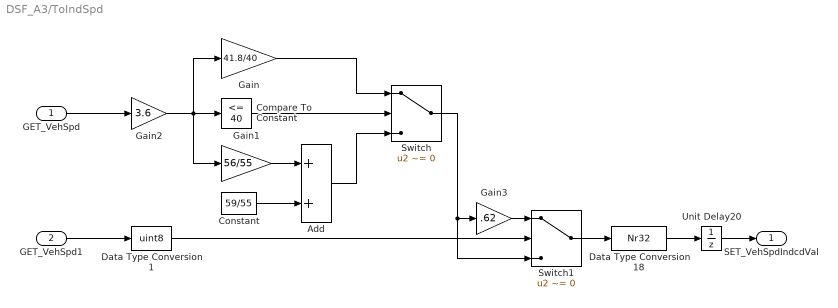
== system DSF_A3/ToIndSpd ==
  GET_VehSpd : Inport
  GET_VehSpd1 : Inport  Port=2
  Add : Sum
  Compare To Constant : simulink/Logic and Bit Operations/Compare To Constant  relop=<=  const=40  OutDataTypeStr=boolean
  Constant : Constant  Value=59/55
  Data Type Conversion1 : DataTypeConversion  OutDataTypeStr=uint8  RndMeth=Round  SaturateOnIntegerOverflow=off
  Data Type Conversion18 : DataTypeConversion  OutDataTypeStr=Nr32  RndMeth=Round  SaturateOnIntegerOverflow=off
  Gain : Gain  Gain=41.8/40
  Gain1 : Gain  Gain=56/55
  Gain2 : Gain  Gain=3.6
  Gain3 : Gain  Gain=.62
  Switch : Switch  Criteria=u2 ~= 0  SaturateOnIntegerOverflow=off  InputSameDT=off
  Switch1 : Switch  Criteria=u2 ~= 0  SaturateOnIntegerOverflow=off  InputSameDT=off
  Unit Delay20 : UnitDelay  InitialCondition=50  SampleTime=-1  HasFrameUpgradeWarning=on
  SET_VehSpdIndcdVal : Outport
  wires:
  GET_VehSpd/1 -> Gain2/1
  Data Type Conversion18/1 -> Unit Delay20/1
  Switch/1 -> Switch1/3, Gain3/1
  Compare To Constant/1 -> Switch/2
  Gain/1 -> Switch/1
  Constant/1 -> Add/2
  Gain1/1 -> Add/1
  Add/1 -> Switch/3
  Gain2/1 -> Gain1/1, Gain/1, Compare To Constant/1
  Unit Delay20/1 -> SET_VehSpdIndcdVal/1
  GET_VehSpd1/1 -> Data Type Conversion1/1
  Switch1/1 -> Data Type Conversion18/1
  Gain3/1 -> Switch1/1
  Data Type Conversion1/1 -> Switch1/2
